simulink model "tesys"  (R2020b)
settings: Solver=ode15s  StartTime=0.0  StopTime=2  RelTol=1e-3  EnableMultiTasking=on
PreLoadFcn:
  | run('C:\users\mazen\source\MATLAB\lib\truetime-2.0\init_truetime');
  | addpath('_tt');
values from neighbouring files (symbols this model uses):
  chisqResidualExp = [0.0306450479532 0.0531264498325 0.923642363871 -0.0297874458631 -0.514662448138 -0.00656924053761 -0.0063391426586 0.00645293061692 -0.0736933231173 -0.060106090774 -0.0130451403889 -0.410405834788 ... (256 elements, 16x16)]    [basevars_performanceTests.mat]
  threshold = 25.9894230826    [basevars_performanceTests.mat]
  u0 = [63.053 53.98 24.644 61.302 22.21 40.064 38.1 46.534 47.446 41.106 18.114 50]    [basevars_performanceTests.mat]
  y0 = [0.250521392428 3664.03885069 4509.26819729 9.3477426267 2704.99998425 74.9999967369 120.399999605 0.337117068415 80.1094039946 50.0000005823 25.1601724781 49.9999996443 ... (16 elements, 16x1)]    [basevars_performanceTests.mat]
undefined symbols (not defined in the file or in its folder): Discrete, ssid_est, ssid_gsp, Time
libraries: truetime x54, ctrlSharedLib x1
settings Model: Creator=ricker  LastModifiedBy=mazen
settings DataIOCC: SaveFinalState=on  SaveFormat=Array  SignalLoggingSaveFormat=ModelDataLogs  SaveOutput=off  SignalLogging=off  DSMLogging=off  SaveTime=off  SignalLoggingName=sigsOut
settings OptimizationCC: LifeSpan=inf
settings DebuggingCC: SaveWithParameterizedLinksMsg=none  UnderspecifiedInitializationDetection=Classic  MergeDetectMultiDrivingBlocksExec=none  SignalResolutionControl=TryResolveAllWithWarning  MultiTaskDSMMsg=warning  MultiTaskCondExecSysMsg=none  SFUnexpectedBacktrackingDiag=warning  SFNoUnconditionalDefaultTransitionDiag=warning  SFExecutionAtInitializationDiag=none  ArithmeticOperatorsInVariantConditions=warning
settings HardwareCC: ProdBitPerPointer=32  ProdBitPerSizeT=32  ProdBitPerPtrDiffT=32  ProdLargestAtomicFloat=None  ProdIntDivRoundTo=Undefined  ProdEndianess=Unspecified  ProdWordSize=32  ProdHWDeviceType=32-bit Generic  TargetUnknown=on
settings ModelReferenceCC: PropagateSignalLabelsOutOfModel=off
settings SFSimCC: SimUseLocalCustomCode=off  CustomCodeUndefinedFunction=UseInterfaceOnly
settings RTWCC: RTWUseLocalCustomCode=off
settings CodeAppCC: StateflowObjectComments=on
settings GRTTargetCC: TargetLangStandard=C89/C90 (ANSI)  CombineOutputUpdateFcns=off  GRTInterface=on
settings ConfigComp: CovMetricSettings=dw  CovSaveCumulativeToWorkspaceVar=on  CovSaveSingleToWorkspaceVar=on  CovExternalEMLEnable=off  CovSFcnEnable=off

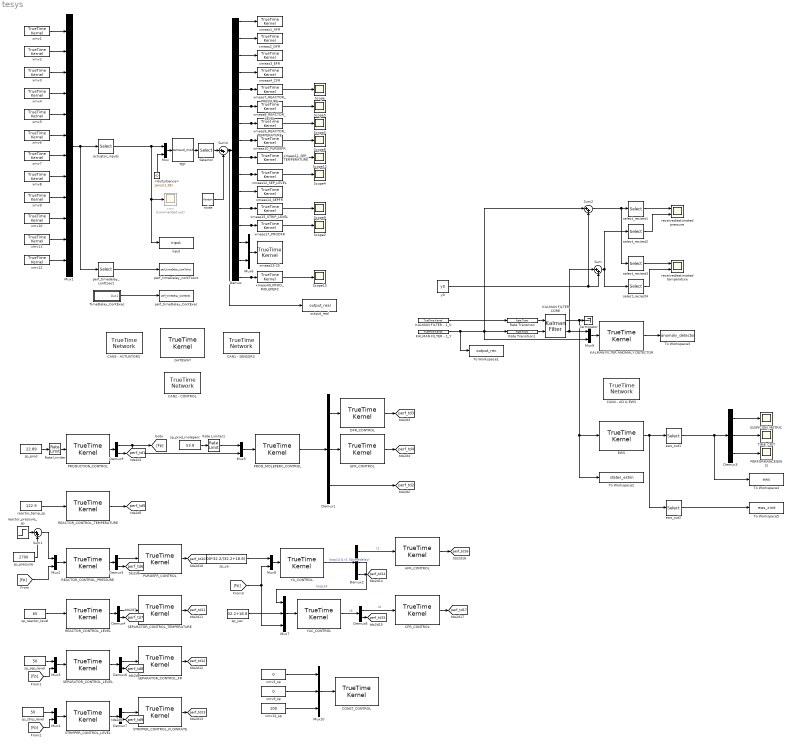
== system tesys ==
  <disturbance> : Constant  Value=zeros(1,28)
  AFR_CONTROL : truetime/TrueTime Kernel  sfun=ctrlvelpi_afr_init  args=[]  ninputsoutputs=[1 1]  ntriggers=0  trigtype=falling  nwnodenbr=[2 17]  clockoffsetdrift=[0 0]  schedoutput=off  battery=off  poweroutput=off  label=2: 17
  CAN1 - SENSORS : truetime/TrueTime Network  nwtype=CSMA/AMP (CAN)  nwnbr=1  nnodes=16  rate=1e9  minsize=8  lossprob=0  seed=0  bandwidths=(1/16)*ones(1,16)  slotsize=512  schedule=[1 1 2]  memsize=80000  buftype=Common buffer  overflow=Retransmit  dynSchedule=0  miniSlotSize=0  NIT=0  QSortMode=FIFO  sync=0  irtSchedule=0  nrtLength=0  nodeGraph=0  scheduleoutput=off
  CAN2 - CONTROL : truetime/TrueTime Network  nwtype=CSMA/AMP (CAN)  nwnbr=2  nnodes=19  rate=1e9  minsize=8  lossprob=0  seed=0  bandwidths=1/19*ones(1,19)  slotsize=512  schedule=[1 1 2]  memsize=80000  buftype=Common buffer  overflow=Retransmit  dynSchedule=0  miniSlotSize=0  NIT=0  QSortMode=FIFO  sync=0  irtSchedule=0  nrtLength=0  nodeGraph=0  scheduleoutput=off
  CAN3 - ACTUATORS : truetime/TrueTime Network  nwtype=CSMA/AMP (CAN)  nwnbr=3  nnodes=13  rate=1e9  minsize=8  lossprob=0  seed=0  bandwidths=1/13*ones(1,13)  slotsize=512  schedule=[1 1 2]  memsize=80000  buftype=Common buffer  overflow=Retransmit  dynSchedule=0  miniSlotSize=0  NIT=0  QSortMode=FIFO  sync=0  irtSchedule=0  nrtLength=0  nodeGraph=0  scheduleoutput=off
  CAN4 - AD & EWS : truetime/TrueTime Network  nwtype=CSMA/AMP (CAN)  nwnbr=4  nnodes=5  rate=5e9  minsize=8  lossprob=0  seed=0  bandwidths=(1/16)*ones(1,16)  slotsize=512  schedule=[1 1 2]  memsize=80000  buftype=Common buffer  overflow=Retransmit  dynSchedule=0  miniSlotSize=0  NIT=0  QSortMode=FIFO  sync=0  irtSchedule=0  nrtLength=0  nodeGraph=0  scheduleoutput=off
  CFR_CONTROL : truetime/TrueTime Kernel  sfun=ctrlvelpi_cfr_init  args=[]  ninputsoutputs=[1 1]  ntriggers=0  trigtype=falling  nwnodenbr=[2 18]  clockoffsetdrift=[0 0]  schedoutput=off  battery=off  poweroutput=off  label=2: 18
  CONST_CONTROL : truetime/TrueTime Kernel  sfun=ctrlconst_init  args=[]  ninputsoutputs=[3 0]  ntriggers=0  trigtype=falling  nwnodenbr=[2 19]  clockoffsetdrift=[0 0]  schedoutput=off  battery=off  poweroutput=off  label=2: 19
  DFR_CONTROL : truetime/TrueTime Kernel  sfun=ctrlvelpi_dfr_init  args=[]  ninputsoutputs=[1 1]  ntriggers=0  trigtype=falling  nwnodenbr=[2 13]  clockoffsetdrift=[0 0]  schedoutput=off  battery=off  poweroutput=off  label=2: 13
  Demux : Demux  Outputs=16
      settings: DisplayOption=none
  Demux1 : Demux  Outputs=3
  Demux2 : Demux  Outputs=3
  Demux3 : Demux  Outputs=3
  Demux{4..9} (6 alike) : Demux  Outputs=2
  EFR_CONTROL : truetime/TrueTime Kernel  sfun=ctrlvelpi_efr_init  args=[]  ninputsoutputs=[1 1]  ntriggers=0  trigtype=falling  nwnodenbr=[2 14]  clockoffsetdrift=[0 0]  schedoutput=off  battery=off  poweroutput=off  label=2: 14
  EWS : truetime/TrueTime Kernel  sfun=ews_init  args=struct('Gsp', ssid_gsp, 'y0', y0, 'u0', u0,'numsteps',500,'Log',1)  ninputsoutputs=[size(ssid_est.A,1), size(ssid_est.A,1)+39+12+3]  ntriggers=0  trigtype=falling  nwnodenbr=[4 5]  clockoffsetdrift=[0 0]  schedoutput=off  battery=off  poweroutput=off  label=4: 5
  GATEWAY : truetime/TrueTime Kernel  sfun=gateway_init  args=[]  ninputsoutputs=[0 0]  ntriggers=0  trigtype=falling  nwnodenbr=[1 1; 2 1; 3 1; 4 1]  clockoffsetdrift=[0 0]  schedoutput=off  battery=off  poweroutput=off  label=1: 1\n2: 1\n3: 1\n4: 1
  KALMAN FILTER ANOMALY DETECTOR : truetime/TrueTime Kernel  sfun=kf2ad_init  args=struct('CovMatrix', chisqResidualExp, 'Threshold', threshold)  ninputsoutputs=[2*16 2]  ntriggers=0  trigtype=falling  nwnodenbr=[4 4]  clockoffsetdrift=[0 0]  schedoutput=off  battery=off  poweroutput=off  label=4: 4
  KALMAN FILTER - 1_U : truetime/TrueTime Kernel  sfun=kf1u_init  args=[]  ninputsoutputs=[0 12]  ntriggers=0  trigtype=falling  nwnodenbr=[4 3]  clockoffsetdrift=[0 0]  schedoutput=off  battery=off  poweroutput=off  label=4: 3
  KALMAN FILTER - 1_Y : truetime/TrueTime Kernel  sfun=kf1y_init  args=struct('y0', y0)  ninputsoutputs=[0 16]  ntriggers=0  trigtype=falling  nwnodenbr=[4 2]  clockoffsetdrift=[0 0]  schedoutput=off  battery=off  poweroutput=off  label=4: 2
  KALMAN FILTER CORE : ctrlSharedLib/Kalman Filter  TimeDomain=Discrete-Time  UseCurrentEstimator=off  ModelSource=LTI State-Space Variable  ModelSourceVariable=ssid_est  A=0.95  B=1  C=1  D=0  NumberOfStates=1  NumberOfInputs=1  NumberOfOutputs=1  InitialEstimateSource=Dialog  X0=0  P0=10  UseK=off  UseGH=off  NumberOfProcessNoiseInputs=1  G=1  TimeInvariantG=on  H=0  TimeInvariantH=on  Q=0.01  TimeInvariantQ=on  R=0.01  TimeInvariantR=on  N=0  TimeInvariantN=on  AddInputPort=on  AddEnablePort=off  OutputEstimatedY=on  OutputP=off  Ts=-1
  Mux{,2..6,8..9} (8 alike) : Mux  Inputs=2
  Mux1 : Mux  Inputs=12
  Mux10 : Mux  Inputs=3
  Mux7 : Mux  Inputs=3
  PERFORMANCE(EWS) : Scope
  PRODUCTION_CONTROL : truetime/TrueTime Kernel  sfun=ctrlvelpiff_production_init  args=[]  ninputsoutputs=[1 2]  ntriggers=0  trigtype=falling  nwnodenbr=[2 4]  clockoffsetdrift=[0 0]  schedoutput=off  battery=off  poweroutput=off  label=2: 4
  PROD_MOLEPERC_CONTROL : truetime/TrueTime Kernel  sfun=ctrlvelpiff_prod_moleperc_init  args=[]  ninputsoutputs=[2 3]  ntriggers=0  trigtype=falling  nwnodenbr=[2 12]  clockoffsetdrift=[0 0]  schedoutput=off  battery=off  poweroutput=off  label=2: 12
  PURGEFR_CONTROL : truetime/TrueTime Kernel  sfun=ctrlvelpi_purgefr_init  args=[]  ninputsoutputs=[1 1]  ntriggers=0  trigtype=falling  nwnodenbr=[2 5]  clockoffsetdrift=[0 0]  schedoutput=off  battery=off  poweroutput=off  label=2: 5
  REACTOR_CONTROL_LEVEL : truetime/TrueTime Kernel  sfun=ctrlvelpi_reactor_level_init  args=[]  ninputsoutputs=[1 2]  ntriggers=0  trigtype=falling  nwnodenbr=[2 6]  clockoffsetdrift=[0 0]  schedoutput=off  battery=off  poweroutput=off  label=2: 6
  REACTOR_CONTROL_PRESSURE : truetime/TrueTime Kernel  sfun=ctrlvelpi_reactor_pressure_init  args=[]  ninputsoutputs=[2 2]  ntriggers=0  trigtype=falling  nwnodenbr=[2 3]  clockoffsetdrift=[0 0]  schedoutput=off  battery=off  poweroutput=off  label=2: 3
  REACTOR_CONTROL_TEMPERATURE : truetime/TrueTime Kernel  sfun=ctrlvelpi_reactor_temperature_init  args=[]  ninputsoutputs=[1 1]  ntriggers=0  trigtype=falling  nwnodenbr=[2 2]  clockoffsetdrift=[0 0]  schedoutput=off  battery=off  poweroutput=off  label=2: 2
  Rate Limiter : RateLimiter  RisingSlewLimit=0.3*22.95/24  FallingSlewLimit=-0.3*22.95/24
  Rate Limiter1 : RateLimiter  RisingSlewLimit=50/24  FallingSlewLimit=-50/24
  Rate Transition : RateTransition  OutPortSampleTime=5e-4
  Rate Transition1 : RateTransition  OutPortSampleTime=5e-4
  SEPARATOR_CONTROL_FR : truetime/TrueTime Kernel  sfun=ctrlvelpi_sepfr_init  args=[]  ninputsoutputs=[1 1]  ntriggers=0  trigtype=falling  nwnodenbr=[2 9]  clockoffsetdrift=[0 0]  schedoutput=off  battery=off  poweroutput=off  label=2: 9
  SEPARATOR_CONTROL_LEVEL : truetime/TrueTime Kernel  sfun=ctrlvelpi_sep_level_init  args=[]  ninputsoutputs=[2 2]  ntriggers=0  trigtype=falling  nwnodenbr=[2 8]  clockoffsetdrift=[0 0]  schedoutput=off  battery=off  poweroutput=off  label=2: 8
  SEPARATOR_CONTROL_TEMPERATURE : truetime/TrueTime Kernel  sfun=ctrlvelpi_sep_temperature_init  args=[]  ninputsoutputs=[1 1]  ntriggers=0  trigtype=falling  nwnodenbr=[2 7]  clockoffsetdrift=[0 0]  schedoutput=off  battery=off  poweroutput=off  label=2: 7
  STRIPPER_CONTROL_FLOWRATE : truetime/TrueTime Kernel  sfun=ctrlvelpi_stripfr_init  args=[]  ninputsoutputs=[1 1]  ntriggers=0  trigtype=falling  nwnodenbr=[2 11]  clockoffsetdrift=[0 0]  schedoutput=off  battery=off  poweroutput=off  label=2: 11
  STRIPPER_CONTROL_LEVEL : truetime/TrueTime Kernel  sfun=ctrlvelpi_strip_level_init  args=[]  ninputsoutputs=[2 2]  ntriggers=0  trigtype=falling  nwnodenbr=[2 10]  clockoffsetdrift=[0 0]  schedoutput=off  battery=off  poweroutput=off  label=2: 10
  SUSPICION_METRIC : Scope
  Scope{,2..5,8..9,12..13} (9 alike) : Scope
  Selector : Selector  InputPortWidth=41  IndexOptions=Index vector (dialog)  Indices=[1:4, 7:12, 14, 15, 17, 23, 25, 40]  OutputSizes=1
  Sum{,1..2,4} (4 alike) : Sum  Inputs=|++
  TEP : S-Function  FunctionName=temexd_mod  Parameters=[], [], 0  SFunctionDeploymentMode=off  EnableBusSupport=off
      mask Display: image('$imagefile'); % Use "Edit Image" on toolstrip to change.
  TIME_CRIT : Scope
  Terminator : Terminator
  TimeDelay_ContExec : Subsystem
  To Workspace1 : ToWorkspace  VariableName=output_rec  SampleTime=0.01
  To Workspace2 : ToWorkspace  VariableName=states_estim  SampleTime=0.01
  To Workspace3 : ToWorkspace  VariableName=anomaly_detector  SampleTime=0.01
  To Workspace4 : ToWorkspace  VariableName=ews  SampleTime=0.01
  To Workspace5 : ToWorkspace  VariableName=ews_xinit  SampleTime=0.01
  YAC_CONTROL : truetime/TrueTime Kernel  sfun=ctrlvelpi_yac_init  args=[]  ninputsoutputs=[3 2]  ntriggers=0  trigtype=falling  nwnodenbr=[2 16]  clockoffsetdrift=[0 0]  schedoutput=off  battery=off  poweroutput=off  label=2: 16
  YA_CONTROL : truetime/TrueTime Kernel  sfun=ctrlvelpi_ya_init  args=[]  ninputsoutputs=[2 3]  ntriggers=0  trigtype=falling  nwnodenbr=[2 15]  clockoffsetdrift=[0 0]  schedoutput=off  battery=off  poweroutput=off  label=2: 15
  actuator_inputs : Selector  InputPortWidth=24  IndexOptions=Index vector (dialog)  Indices=1:2:23  OutputSizes=1
  ews_out1 : Selector  InputPortWidth=size(ssid_est.A,1)+39+12+3  IndexOptions=Index vector (dialog)  Indices=1:3  OutputSizes=1
  ews_out2 : Selector  InputPortWidth=size(ssid_est.A,1)+39+12+3  IndexOptions=Index vector (dialog)  Indices=4:(size(ssid_est.A,1)+39+12+3)  OutputSizes=1
  input : ToWorkspace  VariableName=input  SampleTime=0.01
  noise : RandomNumber  Mean=zeros(16,1)  Variance=0.01*ones(16,1)  SampleTime=5e-4
  output_real : ToWorkspace  VariableName=output_real  SampleTime=0.01
  perf_timeDelay_ContExec : ToWorkspace  VariableName=perf_timeDelay_ContExec  SampleTime=0.01
  perf_timeDelay_contToAct : ToWorkspace  VariableName=perf_timeDelay_contToAct  SampleTime=0.01
  perf_timedelay_conttoact : Selector  InputPortWidth=24  IndexOptions=Index vector (dialog)  Indices=2:2:24  OutputSizes=1
  reactor_pressure_sp : Step  Time=40  After=0  SampleTime=0
  reactor_temp_sp : Constant  Value=122.9
  received/estimated pressure : Scope  NumInputPorts=2
  received/estimated temperature : Scope  NumInputPorts=2
  select_rec/est1 : Selector  InputPortWidth=16  IndexOptions=Index vector (dialog)  Indices=5  OutputSizes=1
  select_rec/est2 : Selector  InputPortWidth=16  IndexOptions=Index vector (dialog)  Indices=5  OutputSizes=1
  select_rec/est3 : Selector  InputPortWidth=16  IndexOptions=Index vector (dialog)  Indices=7  OutputSizes=1
  select_rec/est4 : Selector  InputPortWidth=16  IndexOptions=Index vector (dialog)  Indices=7  OutputSizes=1
  sp_pressure : Constant  Value=2700
  sp_prod : Constant  Value=22.89
  sp_prod_moleperc : Constant  Value=53.8
  sp_reactor_level : Constant  Value=65
  sp_sep_level : Constant  Value=50
  sp_strip_level : Constant  Value=50
  sp_ya : Constant  Value=100*32.2/(32.2+18.8)
  sp_yac : Constant  Value=32.2+18.8
  xmeas10_PURGEFR : truetime/TrueTime Kernel  sfun=sensor_init  args=struct('Name','sensor_purgefr','Ts',5e-4,'Destination',[2 5],'order',8)  ninputsoutputs=[1 0]  ntriggers=0  trigtype=falling  nwnodenbr=[1 4]  clockoffsetdrift=[0 0]  schedoutput=off  battery=off  poweroutput=off  label=1: 4
  xmeas11_SEP_TEMPERATURE : truetime/TrueTime Kernel  sfun=sensor_init  args=struct('Name', 'sensor_sep_temperature', 'Ts', 5e-4, 'Destination', [2 7],'order',9)  ninputsoutputs=[1 0]  ntriggers=0  trigtype=falling  nwnodenbr=[1 7]  clockoffsetdrift=[0 0]  schedoutput=off  battery=off  poweroutput=off  label=1: 7
  xmeas12_SEP_LEVEL : truetime/TrueTime Kernel  sfun=sensor_init  args=struct('Name','sensor_sep_level','Ts',5e-4,'Destination',[2 8],'order',10)  ninputsoutputs=[1 0]  ntriggers=0  trigtype=falling  nwnodenbr=[1 8]  clockoffsetdrift=[0 0]  schedoutput=off  battery=off  poweroutput=off  label=1: 8
  xmeas14_SEPFR : truetime/TrueTime Kernel  sfun=sensor_init  args=struct('Name', 'sensor_sepfr','Ts',5e-4,'Destination', [2 9], 'order', 11)  ninputsoutputs=[1 0]  ntriggers=0  trigtype=falling  nwnodenbr=[1 9]  clockoffsetdrift=[0 0]  schedoutput=off  battery=off  poweroutput=off  label=1: 9
  xmeas15_STRIP_LEVEL : truetime/TrueTime Kernel  sfun=sensor_init  args=struct('Name', 'sensor_strip_level', 'Ts', 5e-4, 'Destination', [2 10],'order',12)  ninputsoutputs=[1 0]  ntriggers=0  trigtype=falling  nwnodenbr=[1 10]  clockoffsetdrift=[0 0]  schedoutput=off  battery=off  poweroutput=off  label=1: 10
  xmeas17_PRODFR : truetime/TrueTime Kernel  sfun=sensor_init  args=struct('Name','sensor_productionfr','Ts',5e-4,'Destination',[2 4; 2 11],'order',13)  ninputsoutputs=[1 0]  ntriggers=0  trigtype=falling  nwnodenbr=[1 5]  clockoffsetdrift=[0 0]  schedoutput=off  battery=off  poweroutput=off  label=1: 5
  xmeas1_AFR : truetime/TrueTime Kernel  sfun=sensor_init  args=struct('Name', 'sensor_xmeas1', 'Ts', 5e-4, 'Destination', [2 17],'order',1)  ninputsoutputs=[1 0]  ntriggers=0  trigtype=falling  nwnodenbr=[1 15]  clockoffsetdrift=[0 0]  schedoutput=off  battery=off  poweroutput=off  label=1: 15
  xmeas23-25 : truetime/TrueTime Kernel  sfun=sensor_xmeas2325_init  args=[]  ninputsoutputs=[2 0]  ntriggers=0  trigtype=falling  nwnodenbr=[1 14]  clockoffsetdrift=[0 0]  schedoutput=off  battery=off  poweroutput=off  label=1: 14
  xmeas2_DFR : truetime/TrueTime Kernel  sfun=sensor_init  args=struct('Name', 'sensor_dfr', 'Ts', 5e-4, 'Destination', [2 13],'order',2)  ninputsoutputs=[1 0]  ntriggers=0  trigtype=falling  nwnodenbr=[1 12]  clockoffsetdrift=[0 0]  schedoutput=off  battery=off  poweroutput=off  label=1: 12
  xmeas3_EFR : truetime/TrueTime Kernel  sfun=sensor_init  args=struct('Name', 'sensor_efr','Ts',5e-4,'Destination',[2 14],'order',3)  ninputsoutputs=[1 0]  ntriggers=0  trigtype=falling  nwnodenbr=[1 13]  clockoffsetdrift=[0 0]  schedoutput=off  battery=off  poweroutput=off  label=1: 13
  xmeas40_PROD_MOLEPERC : truetime/TrueTime Kernel  sfun=sensor_init  args=struct('Name', 'sensor_moleperc_prod','Ts',5e-4,'Destination',[2 12],'order',16)  ninputsoutputs=[1 0]  ntriggers=0  trigtype=falling  nwnodenbr=[1 11]  clockoffsetdrift=[0 0]  schedoutput=off  battery=off  poweroutput=off  label=1: 11
  xmeas4_CFR : truetime/TrueTime Kernel  sfun=sensor_init  args=struct('Name', 'sensor_xmeas4', 'Ts', 5e-4, 'Destination', [2 18],'order',4)  ninputsoutputs=[1 0]  ntriggers=0  trigtype=falling  nwnodenbr=[1 16]  clockoffsetdrift=[0 0]  schedoutput=off  battery=off  poweroutput=off  label=1: 16
  xmeas7_REACTOR_PRESSURE : truetime/TrueTime Kernel  sfun=sensor_init  args=struct('Name','sensor_reactor_pressure','Destination',[2 3],'Ts',5e-4,'order',5)  ninputsoutputs=[1 0]  ntriggers=0  trigtype=falling  nwnodenbr=[1 3]  clockoffsetdrift=[0 0]  schedoutput=off  battery=off  poweroutput=off  label=1: 3
  xmeas8_REACTOR_LEVEL : truetime/TrueTime Kernel  sfun=sensor_init  args=struct('Name', 'sensor_reactor_level', 'Ts', 5e-4, 'Destination', [2 6],'order',6)  ninputsoutputs=[1 0]  ntriggers=0  trigtype=falling  nwnodenbr=[1 6]  clockoffsetdrift=[0 0]  schedoutput=off  battery=off  poweroutput=off  label=1: 6
  xmeas9_REACTOR_TEMPERATURE : truetime/TrueTime Kernel  sfun=sensor_init  args=struct('Destination', [2 2], 'Ts', 5e-4, 'Name', 'sensor_reactor_temperature','order',7)  ninputsoutputs=[1 0]  ntriggers=0  trigtype=falling  nwnodenbr=[1 2]  clockoffsetdrift=[0 0]  schedoutput=off  battery=off  poweroutput=off  label=1: 2
  xmv : Scope  Commented=on
  xmv1 : truetime/TrueTime Kernel  sfun=actuator_init  args=struct('Name', 'actuator_xmv1','x0',63.053)  ninputsoutputs=[0 2]  ntriggers=0  trigtype=falling  nwnodenbr=[3 7]  clockoffsetdrift=[0 0]  schedoutput=off  battery=off  poweroutput=off  label=3: 7
  xmv10 : truetime/TrueTime Kernel  sfun=actuator_init  args=struct('x0', 41.106, 'Name', 'xmv10')  ninputsoutputs=[0 2]  ntriggers=0  trigtype=falling  nwnodenbr=[3 2]  clockoffsetdrift=[0 0]  schedoutput=off  battery=off  poweroutput=off  label=3: 2
  xmv11 : truetime/TrueTime Kernel  sfun=actuator_init  args=struct('Name', 'actuator_xmv11', 'x0', 18.114)  ninputsoutputs=[0 2]  ntriggers=0  trigtype=falling  nwnodenbr=[3 4]  clockoffsetdrift=[0 0]  schedoutput=off  battery=off  poweroutput=off  label=3: 4
  xmv12 : truetime/TrueTime Kernel  sfun=actuator_init  args=struct('x0', 100, 'Name', 'xmv12')  ninputsoutputs=[0 2]  ntriggers=0  trigtype=falling  nwnodenbr=[3 13]  clockoffsetdrift=[0 0]  schedoutput=off  battery=off  poweroutput=off  label=3: 13
  xmv12_sp : Constant  Value=100
  xmv2 : truetime/TrueTime Kernel  sfun=actuator_init  args=struct('Name','actuator_xmv2', 'x0',53.98)  ninputsoutputs=[0 2]  ntriggers=0  trigtype=falling  nwnodenbr=[3 8]  clockoffsetdrift=[0 0]  schedoutput=off  battery=off  poweroutput=off  label=3: 8
  xmv3 : truetime/TrueTime Kernel  sfun=actuator_init  args=struct('Name', 'actuator_xmv3','x0',24.644)  ninputsoutputs=[0 2]  ntriggers=0  trigtype=falling  nwnodenbr=[3 9]  clockoffsetdrift=[0 0]  schedoutput=off  battery=off  poweroutput=off  label=3: 9
  xmv4 : truetime/TrueTime Kernel  sfun=actuator_init  args=struct('Name', 'actuator_xmv4', 'x0', 61.3)  ninputsoutputs=[0 2]  ntriggers=0  trigtype=falling  nwnodenbr=[3 10]  clockoffsetdrift=[0 0]  schedoutput=off  battery=off  poweroutput=off  label=3: 10
  xmv5 : truetime/TrueTime Kernel  sfun=actuator_init  args=struct('x0', 0, 'Name', 'xmv5')  ninputsoutputs=[0 2]  ntriggers=0  trigtype=falling  nwnodenbr=[3 11]  clockoffsetdrift=[0 0]  schedoutput=off  battery=off  poweroutput=off  label=3: 11
  xmv5_sp : Constant  Value=0
  xmv6 : truetime/TrueTime Kernel  sfun=actuator_init  args=struct('Name','actuator_xmv6', 'x0', 40.064)  ninputsoutputs=[0 2]  ntriggers=0  trigtype=falling  nwnodenbr=[3 3]  clockoffsetdrift=[0 0]  schedoutput=off  battery=off  poweroutput=off  label=3: 3
  xmv7 : truetime/TrueTime Kernel  sfun=actuator_init  args=struct('Name','actuator_xmv7','x0',38.1)  ninputsoutputs=[0 2]  ntriggers=0  trigtype=falling  nwnodenbr=[3 5]  clockoffsetdrift=[0 0]  schedoutput=off  battery=off  poweroutput=off  label=3: 5
  xmv8 : truetime/TrueTime Kernel  sfun=actuator_init  args=struct('Name', 'actuator_xmv8', 'x0',46.534)  ninputsoutputs=[0 2]  ntriggers=0  trigtype=falling  nwnodenbr=[3 6]  clockoffsetdrift=[0 0]  schedoutput=off  battery=off  poweroutput=off  label=3: 6
  xmv9 : truetime/TrueTime Kernel  sfun=actuator_init  args=struct('x0', 0, 'Name', 'xmv9')  ninputsoutputs=[0 2]  ntriggers=0  trigtype=falling  nwnodenbr=[3 12]  clockoffsetdrift=[0 0]  schedoutput=off  battery=off  poweroutput=off  label=3: 12
  xmv9_sp : Constant  Value=0
  y0 : Constant  Value=y0
  tag scope: perf_td10=global, perf_td11=global, perf_td12=global, perf_td13=global, perf_td14=global, perf_td15=global, perf_td16=global, perf_td17=global, perf_td1=global, perf_td2=global, perf_td3=global, perf_td4=global, perf_td5=global, perf_td6=global, perf_td7=global, perf_td8=global, perf_td9=global
  wires:
  KALMAN FILTER - 1_U/1 -> Rate Transition/1
  KALMAN FILTER - 1_Y/1 -> To Workspace1/1, Rate Transition1/1, Mux9/2, Sum2/1
  KALMAN FILTER CORE/1 -> To Workspace2/1, EWS/1, Terminator/1
  KALMAN FILTER CORE/2 -> Mux9/1, Sum/1
  Rate Transition/1 -> KALMAN FILTER CORE/1
  Rate Transition1/1 -> KALMAN FILTER CORE/2
  KALMAN FILTER ANOMALY DETECTOR/1 -> To Workspace3/1
  select_rec/est2/1 -> received/estimated pressure/2
  select_rec/est4/1 -> received/estimated temperature/2
  select_rec/est1/1 -> received/estimated pressure/1
  select_rec/est3/1 -> received/estimated temperature/1
  Sum2/1 -> select_rec/est3/1, select_rec/est1/1
  Sum/1 -> select_rec/est4/1, select_rec/est2/1
  y0/1 -> Sum/2, Sum2/2
  Mux9/1 -> KALMAN FILTER ANOMALY DETECTOR/1
  Demux3/1 -> SUSPICION_METRIC/1
  ews_out1/1 -> To Workspace4/1, Demux3/1
  Demux3/3 -> PERFORMANCE(EWS)/1
  Demux3/2 -> TIME_CRIT/1
  Demux4/2 -> [perf_td7]
  Demux1/1 -> DFR_CONTROL/1
  Demux/16 -> xmeas40_PROD_MOLEPERC/1, Scope13/1
  TimeDelay_ContExec/1(Out1) -> perf_timeDelay_ContExec/1
  Mux8/1 -> YA_CONTROL/1
  Demux/2 -> xmeas2_DFR/1
  xmv9_sp/1 -> Mux10/2
  Demux8/2 -> [perf_td15]
  reactor_temp_sp/1 -> REACTOR_CONTROL_TEMPERATURE/1
  Demux2/3 -> [perf_td14]
  PURGEFR_CONTROL/1 -> [perf_td10]
  Demux1/2 -> EFR_CONTROL/1
  Rate Limiter1/1 -> Mux5/1
  CFR_CONTROL/1 -> [perf_td17]
  Demux9/2 -> [perf_td1]
  Mux5/1 -> PROD_MOLEPERC_CONTROL/1
  Demux7/2 -> [perf_td9]
  SEPARATOR_CONTROL_LEVEL/1 -> Demux6/1
  Demux/8 -> Scope8/1, xmeas10_PURGEFR/1
  SEPARATOR_CONTROL_FR/1 -> [perf_td12]
  STRIPPER_CONTROL_FLOWRATE/1 -> [perf_td13]
  [Fp] -> Mux4/2
  Demux/14 -> Mux6/1
  REACTOR_CONTROL_LEVEL/1 -> Demux4/1
  Selector/1 -> Sum4/1
  REACTOR_CONTROL_TEMPERATURE/1 -> [perf_td5]
  Demux/9 -> xmeas11_SEP_TEMPERATURE/1, Scope12/1
  xmv2/1 -> Mux1/2
  AFR_CONTROL/1 -> [perf_td16]
  Demux5/2 -> [perf_td6]
  Mux10/1 -> CONST_CONTROL/1
  xmv6/1 -> Mux1/6
  Demux/11 -> xmeas14_SEPFR/1
  Demux/12 -> xmeas15_STRIP_LEVEL/1, Scope9/1
  PRODUCTION_CONTROL/1 -> Demux9/1
  YAC_CONTROL/1 -> Demux8/1  "r4"
  Demux/3 -> xmeas3_EFR/1
  Demux1/3 -> [perf_td2]
  reactor_pressure_sp/1 -> Sum1/1
  Sum1/1 -> Mux2/1
  [Fp] -> Mux3/2
  Mux1/1 -> perf_timedelay_conttoact/1, actuator_inputs/1
  Sum4/1 -> output_real/1, Demux/1
  [Fp] -> Mux8/2, Mux7/3
  xmv7/1 -> Mux1/7
  Demux/1 -> xmeas1_AFR/1
  REACTOR_CONTROL_PRESSURE/1 -> Demux5/1
  perf_timedelay_conttoact/1 -> perf_timeDelay_contToAct/1
  sp_ya/1 -> Mux8/1
  noise/1 -> Sum4/2
  xmv5_sp/1 -> Mux10/1
  xmv12_sp/1 -> Mux10/3
  xmv5/1 -> Mux1/5
  YA_CONTROL/1 -> Demux2/1  "loop14 & r1 (&timedelay)"
  xmv4/1 -> Mux1/4
  xmv12/1 -> Mux1/12
  Demux2/2 -> Mux7/1  "loop14"
  Demux8/1 -> CFR_CONTROL/1  "r4"
  Demux/4 -> xmeas4_CFR/1
  xmv9/1 -> Mux1/9
  sp_strip_level/1 -> Mux4/1
  sp_reactor_level/1 -> REACTOR_CONTROL_LEVEL/1
  Mux4/1 -> STRIPPER_CONTROL_LEVEL/1
  Mux3/1 -> SEPARATOR_CONTROL_LEVEL/1
  sp_sep_level/1 -> Mux3/1
  Demux/10 -> xmeas12_SEP_LEVEL/1, Scope4/1
  Mux2/1 -> REACTOR_CONTROL_PRESSURE/1
  Demux6/1 -> SEPARATOR_CONTROL_FR/1
  xmv8/1 -> Mux1/8
  Demux6/2 -> [perf_td8]
  xmv1/1 -> Mux1/1
  [Fp] -> Mux2/2
  Demux/15 -> Mux6/2
  sp_pressure/1 -> Sum1/2
  sp_yac/1 -> Mux7/2
  Demux5/1 -> PURGEFR_CONTROL/1
  Mux/1 -> TEP/1
  xmv10/1 -> Mux1/10
  Mux6/1 -> xmeas23-25/1
  Demux/13 -> Scope2/1, xmeas17_PRODFR/1
  Demux4/1 -> SEPARATOR_CONTROL_TEMPERATURE/1
  Rate Limiter/1 -> PRODUCTION_CONTROL/1
  sp_prod/1 -> Rate Limiter/1
  sp_prod_moleperc/1 -> Rate Limiter1/1
  Demux/7 -> Scope3/1, xmeas9_REACTOR_TEMPERATURE/1
  Demux7/1 -> STRIPPER_CONTROL_FLOWRATE/1
  TEP/1 -> Selector/1
  <disturbance>/1 -> Mux/2
  xmv11/1 -> Mux1/11
  Demux/6 -> Scope5/1, xmeas8_REACTOR_LEVEL/1
  DFR_CONTROL/1 -> [perf_td3]
  STRIPPER_CONTROL_LEVEL/1 -> Demux7/1
  Mux7/1 -> YAC_CONTROL/1
  Demux9/1 -> Mux5/2, [Fp]
  Demux/5 -> Scope/1, xmeas7_REACTOR_PRESSURE/1
  EFR_CONTROL/1 -> [perf_td4]
  xmv3/1 -> Mux1/3
  actuator_inputs/1 -> input/1, xmv/1, Mux/1
  PROD_MOLEPERC_CONTROL/1 -> Demux1/1
  SEPARATOR_CONTROL_TEMPERATURE/1 -> [perf_td11]
  Demux2/1 -> AFR_CONTROL/1  "r1"
  EWS/1 -> ews_out2/1, ews_out1/1
  ews_out2/1 -> To Workspace5/1

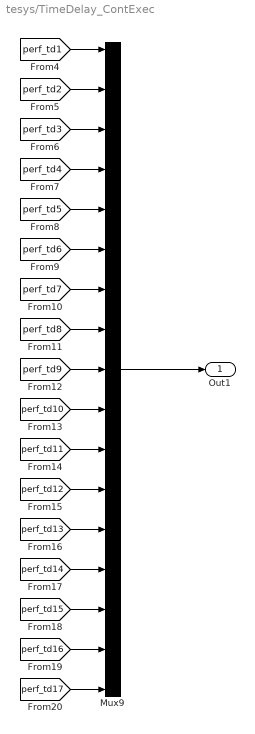
== system tesys/TimeDelay_ContExec ==
  Mux9 : Mux  Inputs=17
  Out1 : Outport
  wires:
  [perf_td15] -> Mux9/15
  [perf_td2] -> Mux9/2
  [perf_td14] -> Mux9/14
  [perf_td3] -> Mux9/3
  [perf_td4] -> Mux9/4
  [perf_td13] -> Mux9/13
  [perf_td1] -> Mux9/1
  [perf_td11] -> Mux9/11
  [perf_td5] -> Mux9/5
  [perf_td7] -> Mux9/7
  [perf_td12] -> Mux9/12
  Mux9/1 -> Out1/1
  [perf_td16] -> Mux9/16
  [perf_td9] -> Mux9/9
  [perf_td8] -> Mux9/8
  [perf_td10] -> Mux9/10
  [perf_td17] -> Mux9/17
  [perf_td6] -> Mux9/6
